simulink model "voltage_droop_03"  (R2020b)
settings: Solver=VariableStepAuto  StartTime=0.0  StopTime=1  RelTol=1e-3
libraries: fl_lib x12, nesl_utility x5
settings Model: Creator=gdudgeon  LastModifiedBy=gdudgeon

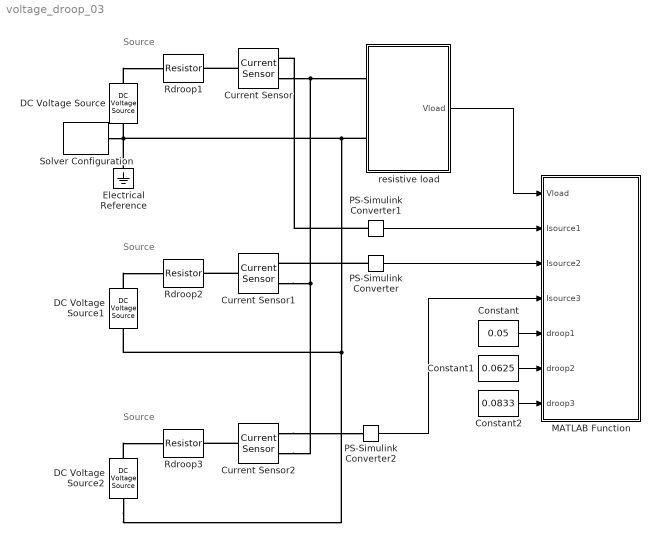
== system voltage_droop_03 ==
  note: Source
  note: Source
  note: Source
  Constant : Constant  Value=0.05
  Constant1 : Constant  Value=0.0625
  Constant2 : Constant  Value=0.0833
  Current Sensor : fl_lib/Electrical/Electrical Sensors/Current Sensor
  Current Sensor1 : fl_lib/Electrical/Electrical Sensors/Current Sensor
  Current Sensor2 : fl_lib/Electrical/Electrical Sensors/Current Sensor
  DC Voltage Source : fl_lib/Electrical/Electrical Sources/DC Voltage Source  v0=1 V
      settings: AttributesFormatString=%<v0>
  DC Voltage Source1 : fl_lib/Electrical/Electrical Sources/DC Voltage Source  v0=1 V
      settings: AttributesFormatString=%<v0>
  DC Voltage Source2 : fl_lib/Electrical/Electrical Sources/DC Voltage Source  v0=1 V
      settings: AttributesFormatString=%<v0>
  Electrical Reference : fl_lib/Electrical/Electrical Elements/Electrical Reference
  MATLAB Function : MATLAB Function  TreatAsAtomicUnit=on  SystemSampleTime=Tanim  mask(Machine Rotor Animation){Tanim=0.01}
      mask prompts: Tanim "Animation Rate [s]"
      mask help: This block animates permanent magnet inside a stator. The "thetaRotor" input is the angle of the rotor. The "phase" parameter must be defined in the workspace and selects the energized coil in the stator.
  PS-Simulink Converter : nesl_utility/PS-Simulink Converter  PhysicalDomain=network_engine_domain  SubClassName=ps_output  LeftPortType=input  RightPortType=output  PseudoPeriodic=off  Frequencies=[]  Unit=inherit  AffineConversion=off
  PS-Simulink Converter1 : nesl_utility/PS-Simulink Converter  PhysicalDomain=network_engine_domain  SubClassName=ps_output  LeftPortType=input  RightPortType=output  PseudoPeriodic=off  Frequencies=[]  Unit=inherit  AffineConversion=off
  PS-Simulink Converter2 : nesl_utility/PS-Simulink Converter  PhysicalDomain=network_engine_domain  SubClassName=ps_output  LeftPortType=input  RightPortType=output  PseudoPeriodic=off  Frequencies=[]  Unit=inherit  AffineConversion=off
  Rdroop1 : fl_lib/Electrical/Electrical Elements/Resistor  R=0.05 Ohm  i_specify=off  i_priority=None  i=0 A  i_nominal_specify=off  i_nominal_unit=A  i_nominal_value=1  v_specify=off  v_priority=None  v=0 V  v_nominal_specify=off  v_nominal_unit=V  v_nominal_value=1
  "Rdroop2 " : fl_lib/Electrical/Electrical Elements/Resistor  R=0.0625 Ohm  i_specify=off  i_priority=None  i=0 A  i_nominal_specify=off  i_nominal_unit=A  i_nominal_value=1  v_specify=off  v_priority=None  v=0 V  v_nominal_specify=off  v_nominal_unit=V  v_nominal_value=1
  Rdroop3 : fl_lib/Electrical/Electrical Elements/Resistor  R=0.0833 Ohm  i_specify=off  i_priority=None  i=0 A  i_nominal_specify=off  i_nominal_unit=A  i_nominal_value=1  v_specify=off  v_priority=None  v=0 V  v_nominal_specify=off  v_nominal_unit=V  v_nominal_value=1
  Solver Configuration : nesl_utility/Solver Configuration  PhysicalDomain=network_engine_domain  SubClassName=solver  LeftPortType=input  RightPortType=generic  Tones=[]  Harmonics=[]  SimulateNoise=off  Profile=off  UseLocalSampling=off  EnableSwitchedLinearOptims=on  FrequencyDomain=off  UseCCode=off  RelTol=0.001  AbsTol=1e-06  MinStep=1e-09  ToWorkspace=off  RevertToSquareIcSolve=off  NumHomotopyIterations=100  PhasorMode=off  PhasorModeNumHarmonics=1  DoDC=off  ResidualTolerance=1e-09  UseLocalSolver=on  LocalSolverChoice=NE_BACKWARD_EULER_ADVANCER  LocalSolverSampleTime=0.001  DoFixedCost=on  MaxNonlinIter=3  MaxModeIter=2  ComputeImpulses=off  ImpulseIterations=2  LinearAlgebra=auto  EquationFormulation=NE_TIME_EF  DelaysMemoryBudget=1024  AutomaticFiltering=on  FilteringTimeConstant=0.001  PartitionStorageMethod=AS_NEEDED  PartitionMemoryBudget=1024  PartitionMethod=ROBUST
  resistive load : Subsystem
  wires:
  resistive load/1(Vload) -> MATLAB Function/1(Vload)
  PS-Simulink Converter1/1 -> MATLAB Function/2(Isource1)
  PS-Simulink Converter/1 -> MATLAB Function/3(Isource2)
  Constant/1 -> MATLAB Function/5(droop1)
  Constant1/1 -> MATLAB Function/6(droop2)
  PS-Simulink Converter2/1 -> MATLAB Function/4(Isource3)
  Constant2/1 -> MATLAB Function/7(droop3)
  connections:
  DC Voltage Source/LConn1 -- Rdroop1/LConn1
  Electrical Reference/LConn1 -- DC Voltage Source2/RConn1 -- DC Voltage Source1/RConn1 -- resistive load/LConn2 -- DC Voltage Source/RConn1 -- Solver Configuration/RConn1
  Current Sensor/RConn2 -- Current Sensor2/RConn2 -- Current Sensor1/RConn2 -- resistive load/LConn1
  DC Voltage Source1/LConn1 -- "Rdroop2 "/LConn1
  Current Sensor/LConn1 -- Rdroop1/RConn1
  Current Sensor1/LConn1 -- "Rdroop2 "/RConn1
  PS-Simulink Converter/LConn1 -- Current Sensor1/RConn1
  PS-Simulink Converter1/LConn1 -- Current Sensor/RConn1
  Current Sensor2/LConn1 -- Rdroop3/RConn1
  DC Voltage Source2/LConn1 -- Rdroop3/LConn1
  Current Sensor2/RConn1 -- PS-Simulink Converter2/LConn1

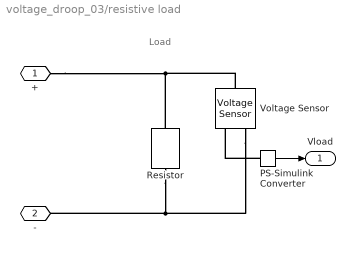
== system voltage_droop_03/resistive load ==
  note: Load
  PS-Simulink Converter : nesl_utility/PS-Simulink Converter  PhysicalDomain=network_engine_domain  SubClassName=ps_output  LeftPortType=input  RightPortType=output  PseudoPeriodic=off  Frequencies=[]  Unit=inherit  AffineConversion=off
  Resistor : fl_lib/Electrical/Electrical Elements/Resistor  R=0.8125 Ohm  i_specify=off  i_priority=None  i=0 A  i_nominal_specify=off  i_nominal_unit=A  i_nominal_value=1  v_specify=off  v_priority=None  v=0 V  v_nominal_specify=off  v_nominal_unit=V  v_nominal_value=1
  Voltage Sensor : fl_lib/Electrical/Electrical Sensors/Voltage Sensor
  + : PMIOPort  Side=Left
  - : PMIOPort  Port=2  Side=Left
  Vload : Outport
  wires:
  PS-Simulink Converter/1 -> Vload/1
  connections:
  PS-Simulink Converter/LConn1 -- Voltage Sensor/RConn1
  Voltage Sensor/RConn2 -- Resistor/RConn1 -- -/RConn1
  Voltage Sensor/LConn1 -- +/RConn1 -- Resistor/LConn1

== matlab function voltage_droop_03/MATLAB Function ==
  data: Vload input; Isource1 input; Isource2 input; Isource3 input; droop1 input; droop2 input; droop3 input
function plotDroop2(Vload,Isource1,Isource2,Isource3,droop1,droop2,droop3)

persistent hf hp hp2 hp3 hp4


if isempty(hf)
    
    figure(1); clf(1); hold on;
    
    [hf,hp,hp2,hp3,hp4] = plotBackground(Vload,Isource1,Isource2,Isource3,droop1,droop2,droop3);
  
    drawnow
    
else
    
    updateAnimation(hp,hp2,hp3,hp4,Vload,Isource1,Isource2,Isource3);

    drawnow

end

end


function [hf,hp,hp2,hp3,hp4] = plotBackground(Vload,Isource1,Isource2,Isource3,droop1,droop2,droop3)

hf = figure(1);hold on,grid %#ok<*DUALC>

hp = plot([0 1],[1 1]*Vload);xlabel('current (A)'),ylabel('Voltage (V)')
hp2 = plot([1 1]*Isource1,[0.91 Vload],'k--');

hp3 = plot([1 1]*Isource2,[0.91 Vload],'k--');

hp4 = plot([1 1]*Isource3,[0.91 Vload],'k--');

plot([0 1],[1 1-droop1],'r');
plot([0 1],[1 1-droop2],'g');
plot([0 1],[1 1-droop3],'b');

coder.extrinsic('num2str')

title(['Droop1 = ',num2str(droop1),' : Droop2 = ',num2str(droop2),' : Droop3 = ',num2str(droop3)])


end

function  updateAnimation(hp,hp2,hp3,hp4,Vload,Isource1,Isource2,Isource3)


set(hp,'YData',[1 1]*Vload);

set(hp2,'XData',[1 1]*Isource1);
set(hp2,'YData',[0.91 Vload]);

set(hp3,'XData',[1 1]*Isource2);
set(hp3,'YData',[0.91 Vload]);

set(hp4,'XData',[1 1]*Isource3);
set(hp4,'YData',[0.91 Vload]);


end
